simulink model "mavsim_show123"  (R2019b)
settings: Solver=ode45  StartTime=0.0  StopTime=300  RelTol=1e-3  EnableMultiTasking=on
InitFcn:
  | param_chap1
undefined symbols (not defined in the file or in its folder): drawEnvironment5, P, path_follow2, path_manager2, path_planner2
settings Model: Creator=beard  LastModifiedBy=liuhan253
settings DataIOCC: LimitDataPoints=on  SaveFormat=Array  SignalLoggingSaveFormat=ModelDataLogs  ReturnWorkspaceOutputs=off
settings OptimizationCC: ExpressionDepthLimit=2147483647  InitFltsAndDblsToZero=on  LifeSpan=inf
settings DebuggingCC: UnderspecifiedInitializationDetection=Classic  MergeDetectMultiDrivingBlocksExec=none  SolverPrmCheckMsg=warning  FcnCallInpInsideContextMsg=warning  AllowSymbolicDim=off  StateNameClashWarn=warning  SFUnexpectedBacktrackingDiag=warning  SFNoUnconditionalDefaultTransitionDiag=warning  SFExecutionAtInitializationDiag=none  ArithmeticOperatorsInVariantConditions=warning
settings HardwareCC: ProdBitPerPointer=32  ProdBitPerSizeT=32  ProdBitPerPtrDiffT=32  ProdLargestAtomicFloat=None  ProdIntDivRoundTo=Undefined  ProdEndianess=Unspecified  ProdWordSize=32  ProdHWDeviceType=32-bit Generic
settings ModelReferenceCC: PropagateSignalLabelsOutOfModel=off
settings SFSimCC: SimUseLocalCustomCode=off  SimParseCustomCode=off  CustomCodeUndefinedFunction=UseInterfaceOnly
settings RTWCC: RTWUseLocalCustomCode=off
settings CodeAppCC: StateflowObjectComments=on
settings GRTTargetCC: TargetLangStandard=C89/C90 (ANSI)  GeneratePreprocessorConditionals=Disable all  CombineOutputUpdateFcns=off  GRTInterface=on
settings ConfigComp: CovMetricSettings=dw  CovHtmlReporting=on  CovSaveCumulativeToWorkspaceVar=on  CovSaveSingleToWorkspaceVar=on  CovExternalEMLEnable=off  CovSFcnEnable=off

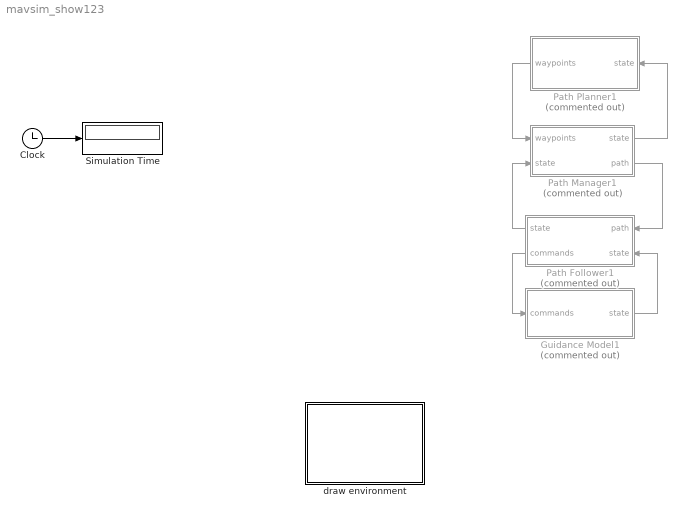
== system mavsim_show123 ==
  Clock : Clock
  Guidance Model1 : Subsystem  Commented=on
  Path Follower1 : Subsystem  Commented=on
  Path Manager1 : Subsystem  Commented=on
  Path Planner1 : Subsystem  Commented=on
  Simulation Time : Display
  draw environment : Subsystem
      mask Display: image(imread('predator.jpg'))
  wires:
  Clock/1 -> Simulation Time/1
  Path Manager1/2(path) -> Path Follower1/1(path)
  Path Follower1/2(commands) -> Guidance Model1/1(commands)
  Path Planner1/1(waypoints) -> Path Manager1/1(waypoints)
  Path Manager1/1("state ") -> Path Planner1/1(state)
  Path Follower1/1("state ") -> Path Manager1/2(state)
  Guidance Model1/1(state) -> Path Follower1/2(state)

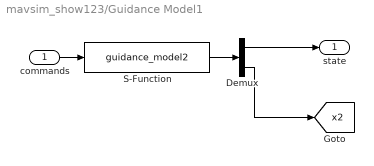
== system mavsim_show123/Guidance Model1 ==
  commands : Inport
  Demux : Demux  Outputs=[16;12]
  S-Function : S-Function  FunctionName=guidance_model2  Parameters=P  SFunctionDeploymentMode=off  EnableBusSupport=off
  state : Outport
  tag scope: x2=global
  wires:
  commands/1 -> S-Function/1
  S-Function/1 -> Demux/1
  Demux/1 -> state/1
  Demux/2 -> [x2]

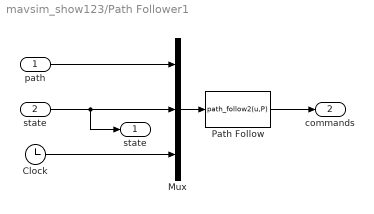
== system mavsim_show123/Path Follower1 ==
  path : Inport
  state : Inport  Port=2
  Clock : Clock
  Mux : Mux  Inputs=3
  Path Follow : MATLABFcn  MATLABFcn=path_follow2(u,P)  OutputDimensions=4  SampleTime=P.Ts
  "state " : Outport
  commands : Outport  Port=2
  wires:
  Path Follow/1 -> commands/1
  Mux/1 -> Path Follow/1
  path/1 -> Mux/1
  Clock/1 -> Mux/3
  state/1 -> Mux/2, "state "/1

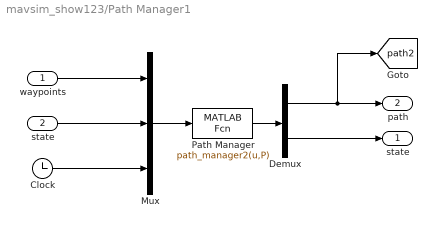
== system mavsim_show123/Path Manager1 ==
  waypoints : Inport
  state : Inport  Port=2
  Clock : Clock
  Demux : Demux  Outputs=[13;17]
  Mux : Mux  Inputs=3
  Path Manager : MATLABFcn  MATLABFcn=path_manager2(u,P)  OutputDimensions=30  SampleTime=P.Ts
  "state " : Outport
  path : Outport  Port=2
  tag scope: path2=global
  wires:
  Demux/2 -> "state "/1
  Demux/1 -> [path2], path/1
  Path Manager/1 -> Demux/1
  waypoints/1 -> Mux/1
  state/1 -> Mux/2
  Clock/1 -> Mux/3
  Mux/1 -> Path Manager/1

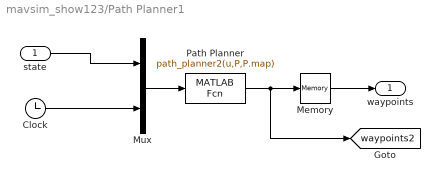
== system mavsim_show123/Path Planner1 ==
  state : Inport
  Clock : Clock
  Memory : Memory
  Mux : Mux  Inputs=2
  Path Planner : MATLABFcn  MATLABFcn=path_planner2(u,P,P.map)  OutputDimensions=1+5*P.size_waypoint_array  SampleTime=100*P.Ts
  waypoints : Outport
  tag scope: waypoints2=global
  wires:
  Mux/1 -> Path Planner/1
  Clock/1 -> Mux/2
  state/1 -> Mux/1
  Path Planner/1 -> Memory/1, [waypoints2]
  Memory/1 -> waypoints/1

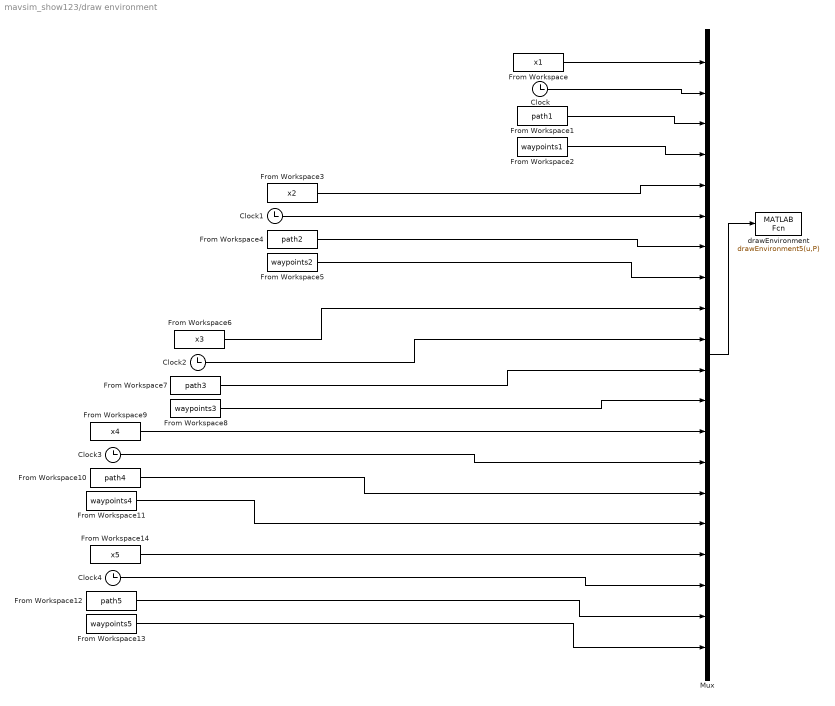
== system mavsim_show123/draw environment ==
  Clock{,1..4} (5 alike) : Clock
  From Workspace : FromWorkspace  VariableName=x1  SampleTime=0.01
  From Workspace1 : FromWorkspace  VariableName=path1  SampleTime=0.01
  From Workspace10 : FromWorkspace  VariableName=path4  SampleTime=0.01
  From Workspace11 : FromWorkspace  VariableName=waypoints4  SampleTime=0.01
  From Workspace12 : FromWorkspace  VariableName=path5  SampleTime=0.01
  From Workspace13 : FromWorkspace  VariableName=waypoints5  SampleTime=0.01
  From Workspace14 : FromWorkspace  VariableName=x5  SampleTime=0.01
  From Workspace2 : FromWorkspace  VariableName=waypoints1  SampleTime=0.01
  From Workspace3 : FromWorkspace  VariableName=x2  SampleTime=0.01
  From Workspace4 : FromWorkspace  VariableName=path2  SampleTime=0.01
  From Workspace5 : FromWorkspace  VariableName=waypoints2  SampleTime=0.01
  From Workspace6 : FromWorkspace  VariableName=x3  SampleTime=0.01
  From Workspace7 : FromWorkspace  VariableName=path3  SampleTime=0.01
  From Workspace8 : FromWorkspace  VariableName=waypoints3  SampleTime=0.01
  From Workspace9 : FromWorkspace  VariableName=x4  SampleTime=0.01
  Mux : Mux  Inputs=20
  drawEnvironment : MATLABFcn  MATLABFcn=drawEnvironment5(u,P)  OutputDimensions=0  SampleTime=0.1
  wires:
  Clock/1 -> Mux/2
  From Workspace/1 -> Mux/1
  Mux/1 -> drawEnvironment/1
  From Workspace1/1 -> Mux/3
  From Workspace2/1 -> Mux/4
  From Workspace4/1 -> Mux/7
  From Workspace5/1 -> Mux/8
  Clock1/1 -> Mux/6
  From Workspace3/1 -> Mux/5
  Clock2/1 -> Mux/10
  From Workspace7/1 -> Mux/11
  From Workspace6/1 -> Mux/9
  From Workspace8/1 -> Mux/12
  Clock3/1 -> Mux/14
  From Workspace9/1 -> Mux/13
  From Workspace10/1 -> Mux/15
  From Workspace11/1 -> Mux/16
  From Workspace13/1 -> Mux/20
  Clock4/1 -> Mux/18
  From Workspace12/1 -> Mux/19
  From Workspace14/1 -> Mux/17
